simulink model "DT_MPC"  (R2025b)
settings: Solver=ode4  StartTime=0.0  StopTime=10  FixedStep=0.01  RelTol=1e-3
model workspace (MAT data in the model file):
  K = 126
  tau = 0.1
libraries: mpclib x1
settings Model: Creator=joshc  LastModifiedBy=joshc

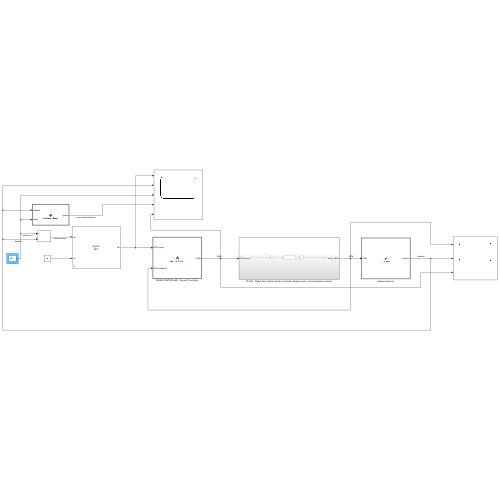
[thumbnail: Simulink's stored preview of the top-level diagram]
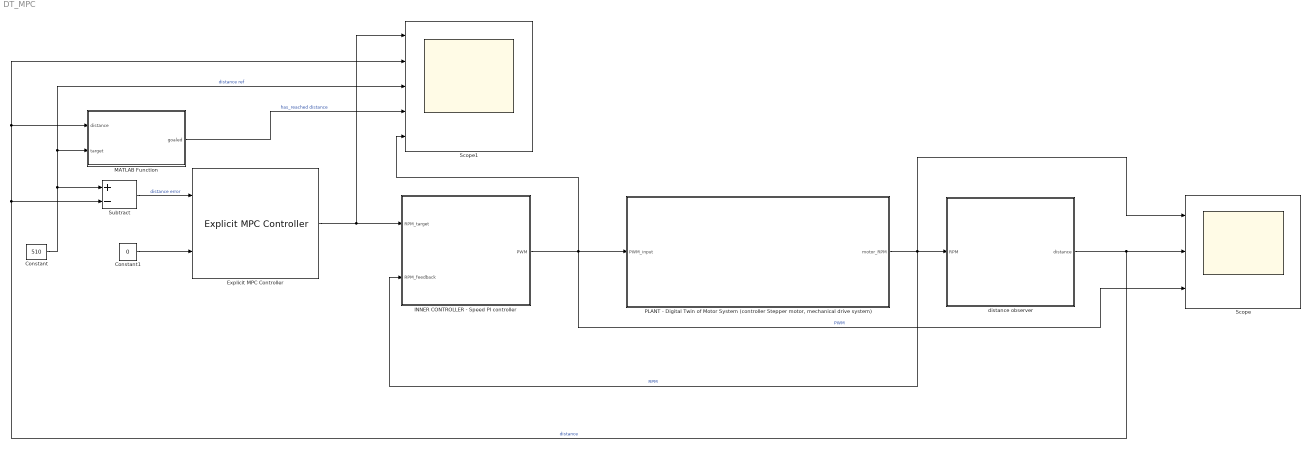
== system DT_MPC ==
  Constant : Constant  Value=510
  Constant1 : Constant  Value=0
  Explicit MPC Controller : mpclib/Explicit MPC Controller  SCDEnableBlockLinearizationSpecification=on  empcobj=explicitMPC  is_multiple=0  enable_value=0  return_u0=off  md_inport=off  mv_inport=off  return_status=off  return_region=off  return_state=off  state_inport=off  BlockDataType=double  SampleTimeInherited=off  switch_inport=off
  INNER CONTROLLER - Speed PI controller : MATLAB Function  TreatAsAtomicUnit=on
  MATLAB Function : MATLAB Function  TreatAsAtomicUnit=on
  "PLANT - Digital Twin of Motor System (controller Stepper motor, mechanical drive system)" : Subsystem
  Scope : Scope  NumInputPorts=3
      settings: ActiveDisplayYMinimum=-3053.6996610955862  ActiveDisplayYMaximum=6636.5388189645846
  Scope1 : Scope  NumInputPorts=5
      settings: ActiveDisplayYMinimum=-126.30597296932822  ActiveDisplayYMaximum=1136.7537567239542
  Subtract : Sum  Inputs=+-
  distance observer : MATLAB Function  TreatAsAtomicUnit=on
  wires:
  INNER CONTROLLER - Speed PI controller/1(PWM) -> Scope1/5, "PLANT - Digital Twin of Motor System (controller Stepper motor, mechanical drive system)"/1(PWM_input), Scope/3  "PWM"
  "PLANT - Digital Twin of Motor System (controller Stepper motor, mechanical drive system)"/1(motor_RPM) -> Scope/1, INNER CONTROLLER - Speed PI controller/2(RPM_feedback), distance observer/1(RPM)  "RPM"
  distance observer/1(distance) -> Subtract/2, MATLAB Function/1(distance), Scope1/2, Scope/2  "distance"
  Explicit MPC Controller/1 -> Scope1/1, INNER CONTROLLER - Speed PI controller/1(RPM_target)
  Constant/1 -> Subtract/1, MATLAB Function/2(target), Scope1/3  "distance ref"
  MATLAB Function/1(goaled) -> Scope1/4  "has_reached distance"
  Subtract/1 -> Explicit MPC Controller/1  "distance error"
  Constant1/1 -> Explicit MPC Controller/2

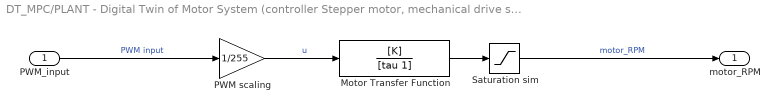
== system DT_MPC/PLANT - Digital Twin of Motor System (controller Stepper motor, mechanical drive system) ==
  PWM_input : Inport
  Motor Transfer Function : TransferFcn  Numerator=[K]  Denominator=[tau 1]
  PWM scaling : Gain  Gain=1/255
  Saturation sim : Saturate  UpperLimit=186  LowerLimit=0
  motor_RPM : Outport
  wires:
  PWM_input/1 -> PWM scaling/1  "PWM input"
  PWM scaling/1 -> Motor Transfer Function/1  "u"
  Motor Transfer Function/1 -> Saturation sim/1
  Saturation sim/1 -> motor_RPM/1  "motor_RPM"

== matlab function DT_MPC/INNER CONTROLLER - Speed PI controller ==
  settings: updateMethod=DISCRETE
  data: RPM_target input; PWM output; RPM_feedback input
function PWM = pid_controller(RPM_target, RPM_feedback)

Kp = 6;
Ki = 0.002;
Kd = 0.0;
Ts = 0.01;

persistent integral prev_error
if isempty(integral)
    integral = 0;
end

if isempty(prev_error)
    prev_error = 0;
end

error = (RPM_target - RPM_feedback);
integral = integral + error*Ts;
derivative = (error - prev_error);

u = Kp*error + Ki*integral + Kd*derivative;
PWM = min(max(u, 0), 255);

prev_error = error;
end

== matlab function DT_MPC/MATLAB Function ==
  data: distance input; goaled output; target input
function goaled = distance_check(distance, target)

if distance >= target - (target/200)
    goaled = 100;
else
    goaled = 0;
end

== matlab function DT_MPC/distance observer ==
  settings: updateMethod=DISCRETE
  data: RPM input; distance output
function distance = rpm2dist(RPM)

diameter = 49.7;
Ts = 0.01;

circumference = pi*diameter;

persistent x
if isempty(x)
    x = 0;
end

speed = (RPM/60)*circumference;

x = x + speed*Ts;

distance = x;
